simulink model "ChrgCtrl"  (R2023a)
settings: Solver=FixedStepDiscrete  StartTime=0.0  StopTime=10  FixedStep=0.01  RelTol=1e-3
model workspace (MAT data in the model file):
  Cal_TrqMax = Simulink.Parameter
  Cal_TrqMax.Value = 1500
  Cal_TrqMax.DataType = 'single'
  Cal_TrqMax.Min = 0
  Cal_TrqMax.Max = 2000
  Cal_TrqMax.Complexity = 'real'
  Cal_TrqMax.Dimensions = [1 1]
  Cal_TrqRate = Simulink.Parameter
  Cal_TrqRate.Value = 2000
  Cal_TrqRate.DataType = 'single'
  Cal_TrqRate.Min = 0
  Cal_TrqRate.Max = 5000
  Cal_TrqRate.Complexity = 'real'
  Cal_TrqRate.Dimensions = [1 1]
undefined symbols (not defined in the file): En_DrvMode
settings Model: Creator=Henry  LastModifiedBy=Henry
settings OptimizationCC: DefaultParameterBehavior=Inlined  EnhancedBackFolding=on  PassReuseOutputArgsAs=Individual arguments  ZeroExternalMemoryAtStartup=off  OptimizeBlockOrder=speed  DifferentSizesBufferReuse=on  OptimizationCustomize=off  EfficientTunableParamExpr=on
settings DebuggingCC: ParameterTunabilityLossMsg=error
settings SFSimCC: MATLABDynamicMemAlloc=off
settings RTWCC: Description=AUTOSAR  SystemTargetFile=autosar.tlc  GenCodeOnly=on  TemplateMakefile=ert_default_tmf  GenerateReport=on
settings CodeAppCC: ForceParamTrailComments=on  IgnoreCustomStorageClasses=off  OperatorAnnotations=on  SimulinkDataObjDesc=on  SFDataObjDesc=on  InsertBlockDesc=on
settings STFCustomTargetCC: MultiwordLength=256  ParMdlRefBuildCompliant=on  CompOptLevelCompliant=on  ConcurrentExecutionCompliant=off  IncludeMdlTerminateFcn=off  CombineOutputUpdateFcns=on  SuppressErrorStatus=on  ERTCustomFileBanners=on  CodeInterfacePackaging=Reusable function  SupportNonFinite=off  SupportComplex=off  SupportContinuousTime=off  SupportNonInlinedSFcns=off  RemoveResetFunc=on  MATLABClassNameForMDSCustomization=Simulink.SoftwareTarget.ERTCustomization  AutosarCompliant=on  GRTInterface=off  LookupTableObjectStructAxisOrder=2,1,3,4,...  LUTObjectStructOrderEvenSpacing=Size,Table,Breakpoints  SystemTargetFile=autosar.tlc
settings ERTTargetCC: TargetLangStandard=C99 (ISO)  ConcurrentExecutionCompliant=off  IncludeMdlTerminateFcn=off  SuppressErrorStatus=on  CodeInterfacePackaging=Reusable function  SupportNonFinite=off  SupportComplex=off  ModelStepFunctionPrototypeControlCompliant=off  CPPClassGenCompliant=off  AutosarCompliant=on  LookupTableObjectStructAxisOrder=2,1,3,4,...  LUTObjectStructOrderEvenSpacing=Size,Table,Breakpoints  InlinedParameterPlacement=NonHierarchical  ERTCustomFileTemplate=example_file_process.tlc

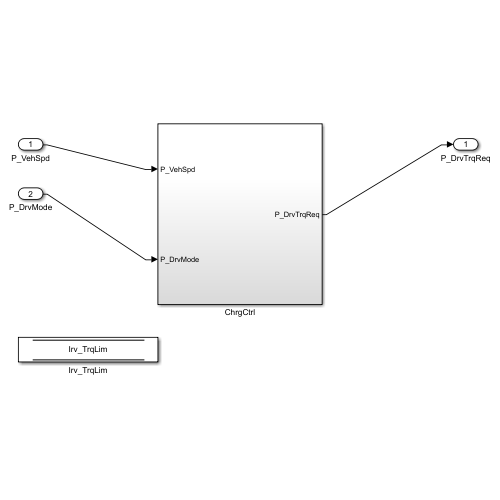
[thumbnail: Simulink's stored preview of the top-level diagram]
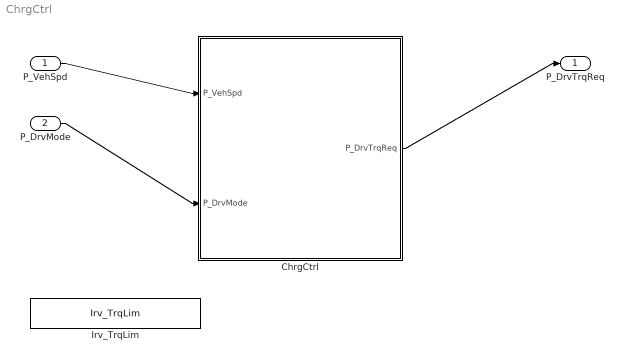
== system ChrgCtrl ==
  P_VehSpd : Inport  OutDataTypeStr=single
  P_DrvMode : Inport  Port=2  OutDataTypeStr=Enum: En_DrvMode
  ChrgCtrl : Subsystem
  Irv_TrqLim : DataStoreMemory  DataStoreName=Irv_TrqLim  WriteAfterWriteMsg=warning  ShowAdditionalParam=off  OutDataTypeStr=single
  P_DrvTrqReq : Outport  OutDataTypeStr=single
  wires:
  P_VehSpd/1 -> ChrgCtrl/1(P_VehSpd)
  P_DrvMode/1 -> ChrgCtrl/2(P_DrvMode)
  ChrgCtrl/1(P_DrvTrqReq) -> P_DrvTrqReq/1

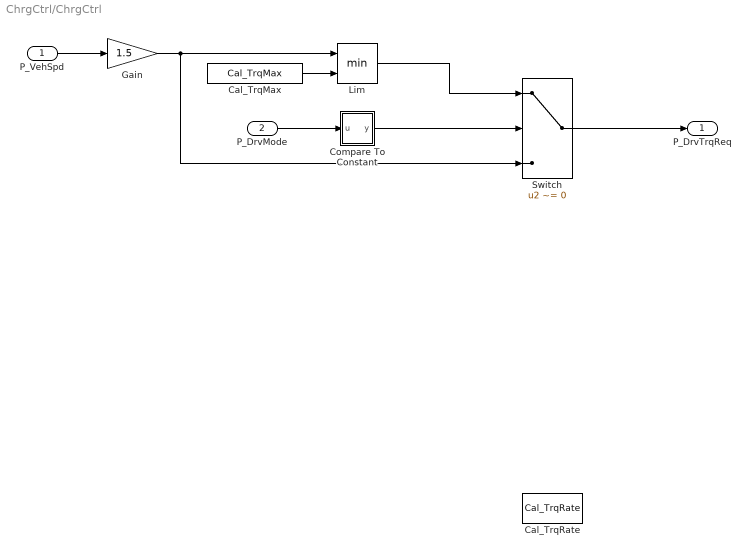
== system ChrgCtrl/ChrgCtrl ==
  P_VehSpd : Inport
  P_DrvMode : Inport  Port=2
  Cal_TrqMax : Constant  Value=Cal_TrqMax
  Cal_TrqRate : Constant  Value=Cal_TrqRate  OutDataTypeStr=single
  Compare To Constant : Subsystem  mask(Compare To Constant){relop===, const=2, OutDataTypeStr=boolean, ZeroCross=on}
      mask prompts: relop "Simulink:masks:Operator_MP"; const "Simulink:masks:ConstantValue_MP"; OutDataTypeStr "Simulink:masks:OutputDataType_MP"; ZeroCross "Simulink:masks:EnableZerocrossingDetection_MP"
      mask help: Simulink:masks:CompareToConstant_MD
      mask init:
      | blkName = gcb;
      | 
      | if strcmp(get_param(gcbh,'OutDataTypeStr'),'boolean')
      | 	setValue = 'boolean';
      | else
      | 	setValue = 'fixdt(0, 8, 0)';
      | end
      | 
      | set_param([blkName,'/Compare'],'relop',relop, ...
      | 	'OutDataTypeStr', setValue, 'ZeroCross', ZeroCross);
      | 
      | str = [relop,' C']; %default
      | 
      | const_str = get_param(blkName, 'const');
      | const_val = str2num(const_str);
      | 
      | if isempty(const_val) %#ok<ST2NM>
      |     %Expression/Variable
      |     str = [relop, ' ', strtrim(const_str)];
      | else
      |     if length(const_val) == 1 
      |         if Simulink.data.isSupportedEnumClass(class(const_val))
      |             % Special Handling for Enumerations
      |             if Simulink.data.getEnumTypeInfo(class(const_val), 'AddClassNameToEnumNames')
      |                 str = [relop, ' ', strtrim(const_str)];
      |             else
      |                 str = [relop, ' ', char(const_val)];
      |             end
      |         elseif(isfloat(const_val) || isinteger(const_val) || islogical(const_val)) 
      |                 str = [relop, ' ', num2str(const_val)];
      |         end
      |     end
      | end
      settings: LibrarySourceBlock=|
      | simulink/Logic and Bit
      | Operations/Compare
      | To Constant
      mask TypeOptions relop: == | ~= | < | <= | >= | >
      mask TypeOptions OutDataTypeStr: Simulink:masks:uint8 | Simulink:masks:boolean
      mask Callback ZeroCross: sl('zeroCrossEnable', gcbh);
      mask Display: disp(str)
  Gain : Gain  Gain=1.5  OutDataTypeStr=single
  Lim : MinMax  Inputs=2  OutDataTypeStr=single
  Switch : Switch  Criteria=u2 ~= 0  OutDataTypeStr=single  SaturateOnIntegerOverflow=off  InputSameDT=off
  P_DrvTrqReq : Outport
  wires:
  Switch/1 -> P_DrvTrqReq/1
  Lim/1 -> Switch/1
  Compare To Constant/1(y) -> Switch/2
  P_DrvMode/1 -> Compare To Constant/1(u)
  P_VehSpd/1 -> Gain/1
  Cal_TrqMax/1 -> Lim/2
  Gain/1 -> Lim/1, Switch/3

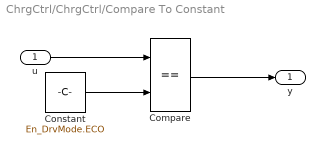
== system ChrgCtrl/ChrgCtrl/Compare To Constant ==
  u : Inport
  Compare : RelationalOperator  Operator===  OutDataTypeStr=boolean
  Constant : Constant  DisableCoverage=on  Value=En_DrvMode.ECO  OutDataTypeStr=Enum: En_DrvMode
  y : Outport
  wires:
  Compare/1 -> y/1
  Constant/1 -> Compare/2
  u/1 -> Compare/1
